simulink model "TestSFC"  (R2013b)
settings: Solver=ode45  StartTime=0.0  StopTime=10.0  RelTol=1e-3
libraries: Lib_Turbo_SFCCalc_TMATS x1
settings Model: Creator=tlavelle  LastModifiedBy=jwchapm2
settings OptimizationCC: ExpressionDepthLimit=2147483647
settings DebuggingCC: StateNameClashWarn=warning

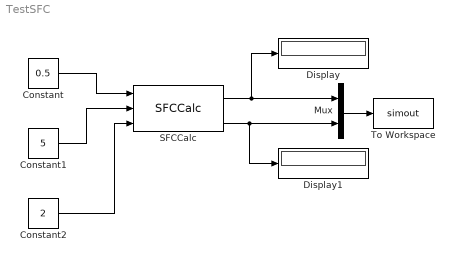
== system TestSFC ==
  Constant : Constant  Value=0.5
  Constant1 : Constant  Value=5
  Constant2 : Constant  Value=2
  Display : Display
  Display1 : Display
  Mux : Mux  Inputs=2
  SFCCalc : Lib_Turbo_SFCCalc_TMATS/SFCCalc
  To Workspace : ToWorkspace  VariableName=simout  SampleTime=-1  SaveFormat=Timeseries
  wires:
  SFCCalc/1 -> Display/1, Mux/1
  SFCCalc/2 -> Display1/1, Mux/2
  Mux/1 -> To Workspace/1
  Constant/1 -> SFCCalc/1
  Constant1/1 -> SFCCalc/2
  Constant2/1 -> SFCCalc/3
